simulink model "InertiaWheelSystem"
settings: Solver=ode45  StartTime=0.0  StopTime=10.0  RelTol=1e-6
values from neighbouring files (symbols this model uses):
  A = [0 1 0; a/Jw 0 0 ; -(a/Jp) 0 0]    [modelFLAWED.m]
  B = [B_tau B_d]    [modelFLAWED.m]
  C = [1 0 0]    [modelFLAWED.m]
  D = 0    [modelFLAWED.m]
undefined symbols (not defined in the file or in its folder): ki, Kt, N, Tdt, Tit, x10, x20, x30
libraries: simulink x5, cstblocks x2
settings Model: Creator=elt11jke  LastModifiedBy=frt090_B
settings DataIOCC: LimitDataPoints=on  SaveFormat=Array  SignalLoggingSaveFormat=ModelDataLogs  ReturnWorkspaceOutputs=off
settings OptimizationCC: ExpressionDepthLimit=2147483647  LifeSpan=inf  SimCompilerOptimization=Off
settings DebuggingCC: UnderspecifiedInitializationDetection=Classic  MergeDetectMultiDrivingBlocksExec=none  SolverPrmCheckMsg=warning  MultiTaskDSMMsg=warning  MultiTaskCondExecSysMsg=none  FcnCallInpInsideContextMsg=Enable All  FrameProcessingCompatibilityMsg=warning  StateNameClashWarn=warning  StrictBusMsg=None  SFUnexpectedBacktrackingDiag=warning  SFNoUnconditionalDefaultTransitionDiag=warning
settings HardwareCC: ProdBitPerPointer=32  ProdLargestAtomicFloat=None  ProdIntDivRoundTo=Undefined  ProdEndianess=Unspecified  ProdWordSize=32  ProdHWDeviceType=32-bit Generic
settings ModelReferenceCC: PropagateSignalLabelsOutOfModel=off
settings SFSimCC: SimUseLocalCustomCode=off
settings RTWCC: RTWUseLocalCustomCode=off  IncludeERTFirstTime=on  RTWCompilerOptimization=Off
settings GRTTargetCC: GeneratePreprocessorConditionals=Disable all

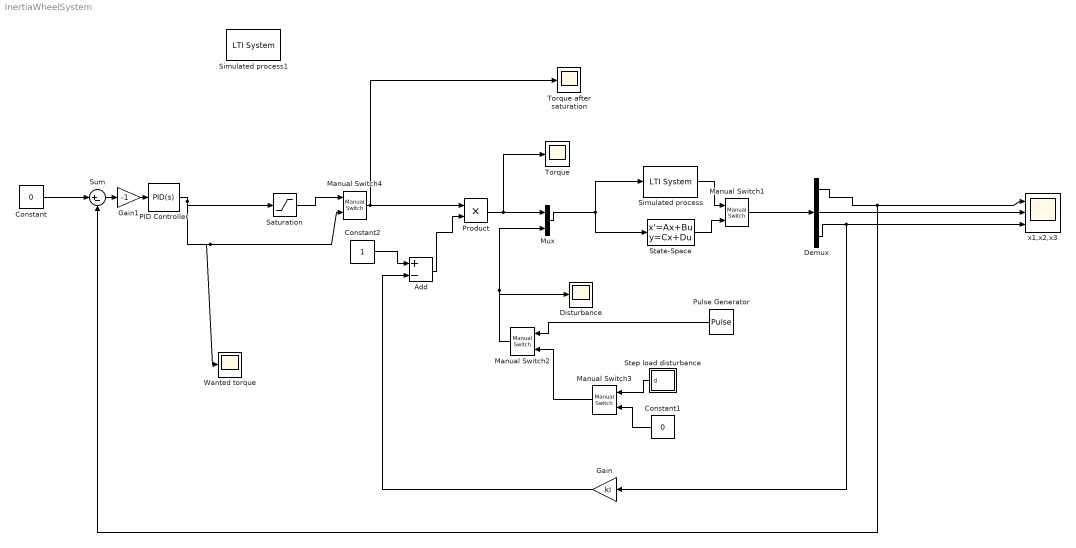
== system InertiaWheelSystem ==
  Add : Sum  Inputs=+-
  Constant : Constant  Value=0
  Constant1 : Constant  Value=0
  Constant2 : Constant
  Demux : Demux  Outputs=3
  Disturbance : Scope
      settings: ShowLegends=on  TimeRange=10  YMin=-0.01  YMax=0.02  SaveName=ScopeData2
  Gain : Gain  Gain=ki
  Gain1 : Gain  Gain=-1
  Manual Switch1 : simulink/Signal Routing/Manual Switch  sw=0  action=0  varsize=off
  Manual Switch2 : simulink/Signal Routing/Manual Switch  sw=0  action=0  varsize=off
  Manual Switch3 : simulink/Signal Routing/Manual Switch  sw=0  action=0  varsize=off
  Manual Switch4 : simulink/Signal Routing/Manual Switch  sw=1  action=0  varsize=off
  Mux : Mux  Inputs=2
  PID Controller : simulink/Continuous/PID Controller  Controller=PID  TimeDomain=Continuous-time  SampleTime=1  IntegratorMethod=Forward Euler  FilterMethod=Forward Euler  Form=Parallel  P=Kt  I=Tit  D=Tdt  N=N  InitialConditionSource=internal  InitialConditionForIntegrator=0  InitialConditionForFilter=0  ExternalReset=none  LimitOutput=off  UpperSaturationLimit=inf  LowerSaturationLimit=-inf  LinearizeAsGain=off  AntiWindupMode=none  Kb=1  TrackingMode=off  Kt=1  PParamMin=[]  PParamMax=[]  IParamMin=[]  IParamMax=[]  DParamMin=[]  DParamMax=[]  NParamMin=[]  NParamMax=[]  KbParamMin=[]  KbParamMax=[]  KtParamMin=[]  KtParamMax=[]  POutMin=[]  POutMax=[]  IOutMin=[]  IOutMax=[]  DOutMin=[]  DOutMax=[]  NOutMin=[]  NOutMax=[]  KbOutMin=[]  KbOutMax=[]  KtOutMin=[]  KtOutMax=[]  IntegratorOutMin=[]  IntegratorOutMax=[]  FilterOutMin=[]  FilterOutMax=[]  SumOutMin=[]  SumOutMax=[]  SumI1OutMin=[]  SumI1OutMax=[]  SumI2OutMin=[]  SumI2OutMax=[]  SumI3OutMin=[]  SumI3OutMax=[]  SumDOutMin=[]  SumDOutMax=[]  SaturationOutMin=[]  SaturationOutMax=[]  IntegratorContinuousStateAttributes=''  IntegratorStateMustResolveToSignalObject=off  IntegratorRTWStateStorageClass=Auto  FilterContinuousStateAttributes=''  FilterStateMustResolveToSignalObject=off  FilterRTWStateStorageClass=Auto
  Product : Product  RndMeth=Zero
  Pulse Generator : DiscretePulseGenerator  PulseType=Time based  Amplitude=0.01  Period=3  PulseWidth=5
  Saturation : Saturate  UpperLimit=0.384  LowerLimit=-0.384
  Simulated process : cstblocks/LTI System  sys=PinSF  IC=[]
  Simulated process1 : cstblocks/LTI System  sys=Cin  IC=[]
  State-Space : StateSpace  A=A  B=B  C=C  D=D  X0=[x10 x20 x30]
  Step load disturbance : Subsystem
  Sum : Sum  Inputs=|+-
  Torque : Scope
      settings: ShowLegends=on  TimeRange=10  YMin=0.3  YMax=0.4
  Torque after saturation : Scope
      settings: ShowLegends=on  TimeRange=10  YMin=0.3648  YMax=0.4032  SaveName=ScopeData4
  Wanted torque : Scope
      settings: ShowLegends=on  TimeRange=10  YMin=-1.355e+07  YMax=-1.3275e+07  SaveName=ScopeData3
  x1,x2,x3 : Scope  NumInputPorts=3
      settings: ShowLegends=on  TimeRange=10  YMin=1000~0~-0.0003  YMax=10000~90000~-2.5e-05
  wires:
  Constant/1 -> Sum/1
  Demux/1 -> x1,x2,x3/1, Sum/2
  Demux/2 -> x1,x2,x3/2
  Pulse Generator/1 -> Manual Switch2/1
  Mux/1 -> State-Space/1, Simulated process/1
  Manual Switch1/1 -> Demux/1
  Step load disturbance/1(d) -> Manual Switch3/1
  Constant1/1 -> Manual Switch3/2
  Manual Switch3/1 -> Manual Switch2/2
  Simulated process/1 -> Manual Switch1/1
  State-Space/1 -> Manual Switch1/2
  Demux/3 -> x1,x2,x3/3, Gain/1
  Gain/1 -> Add/2
  Manual Switch4/1 -> Torque after saturation/1, Product/1
  Constant2/1 -> Add/1
  Add/1 -> Product/2
  Product/1 -> Mux/1, Torque/1
  PID Controller/1 -> Manual Switch4/2, Wanted torque/1, Saturation/1
  Manual Switch2/1 -> Mux/2, Disturbance/1
  Sum/1 -> Gain1/1
  Gain1/1 -> PID Controller/1
  Saturation/1 -> Manual Switch4/1

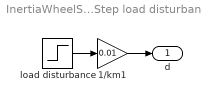
== system InertiaWheelSystem/Step load disturbance ==
  1/km1 : Gain  Gain=0.01  SaturateOnIntegerOverflow=on  OutDataTypeStr=Inherit: Same as input  ParamDataTypeStr=Inherit: Same as input
  load disturbance : Step  Time=5  After=-0.15  SampleTime=0
  d : Outport
  wires:
  load disturbance/1 -> 1/km1/1
  1/km1/1 -> d/1
